simulink library "origionalPlant_cl"  (R2018b)
settings: Solver=VariableStepAuto  StartTime=0.0  StopTime=10.0  RelTol=1e-3
undefined symbols (not defined in the file or in its folder): X0
libraries: winch_ul x1
settings Model: Creator=mcobb  LastModifiedBy=mcobb

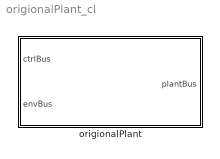
== system origionalPlant_cl ==
  origionalPlant : Subsystem  VariantControl=VSS_plant_origionalPlant

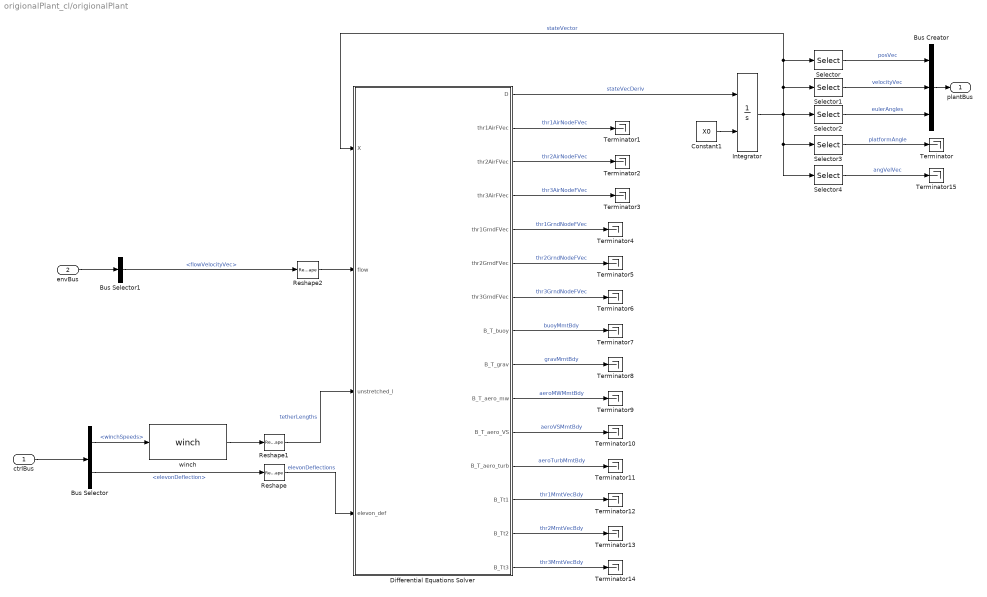
== system origionalPlant_cl/origionalPlant ==
  ctrlBus : Inport  OutDataTypeStr=Bus: ctrlBus
  envBus : Inport  Port=2  OutDataTypeStr=Bus: envBus
  Bus Creator : BusCreator  Inputs=3
  Bus Selector : BusSelector  OutputSignals=winchSpeeds,elevonDeflection
  Bus Selector1 : BusSelector  OutputSignals=flowVelocityVec
  Constant1 : Constant  Value=X0
  Differential Equations Solver : MATLAB Function  TreatAsAtomicUnit=on
  Integrator : Integrator  InitialConditionSource=external  InitialCondition=X0
  Reshape : Reshape  OutputDimensionality=Column vector (2-D)
  Reshape1 : Reshape  OutputDimensionality=Column vector (2-D)
  Reshape2 : Reshape  OutputDimensionality=Column vector (2-D)
  Selector : Selector  InputPortWidth=length(X0)  IndexOptions=Index vector (dialog)  Indices=[1 2 3]  OutputSizes=1
  Selector1 : Selector  InputPortWidth=length(X0)  IndexOptions=Index vector (dialog)  Indices=[4 5 6]  OutputSizes=1
  Selector2 : Selector  InputPortWidth=length(X0)  IndexOptions=Index vector (dialog)  Indices=[7 8 9]  OutputSizes=1
  Selector3 : Selector  InputPortWidth=length(X0)  IndexOptions=Index vector (dialog)  Indices=13  OutputSizes=1
  Selector4 : Selector  InputPortWidth=length(X0)  IndexOptions=Index vector (dialog)  Indices=[10 11 12]  OutputSizes=1
  Terminator{,1..15} (16 alike) : Terminator
  winch : winch_ul/winch  initLength=0  maxSpd=1  tau=0  maxAccl=1
  plantBus : Outport
  wires:
  Bus Selector/2 -> Reshape/1  "<elevonDeflection>"
  Bus Selector/1 -> winch/1  "<winchSpeeds>"
  Constant1/1 -> Integrator/2
  Differential Equations Solver/1(D) -> Integrator/1  "stateVecDeriv"
  Integrator/1 -> Differential Equations Solver/1(X), Selector/1, Selector1/1, Selector4/1, Selector3/1, Selector2/1  "stateVector"
  Selector1/1 -> Bus Creator/2  "velocityVec"
  Selector2/1 -> Bus Creator/3  "eulerAngles"
  Selector/1 -> Bus Creator/1  "posVec"
  Selector3/1 -> Terminator/1  "platformAngle"
  winch/1 -> Reshape1/1
  ctrlBus/1 -> Bus Selector/1
  envBus/1 -> Bus Selector1/1
  Bus Creator/1 -> plantBus/1
  Bus Selector1/1 -> Reshape2/1  "<flowVelocityVec>"
  Reshape/1 -> Differential Equations Solver/4(elevon_def)  "elevonDeflections"
  Reshape1/1 -> Differential Equations Solver/3(unstretched_l)  "tetherLengths"
  Reshape2/1 -> Differential Equations Solver/2(flow)
  Differential Equations Solver/2(thr1AirFVec) -> Terminator1/1  "thr1AirNodeFVec"
  Differential Equations Solver/7(thr3GrndFVec) -> Terminator6/1  "thr3GrndNodeFVec"
  Differential Equations Solver/6(thr2GrndFVec) -> Terminator5/1  "thr2GrndNodeFVec"
  Differential Equations Solver/5(thr1GrndFVec) -> Terminator4/1  "thr1GrndNodeFVec"
  Differential Equations Solver/4(thr3AirFVec) -> Terminator3/1  "thr3AirNodeFVec"
  Differential Equations Solver/3(thr2AirFVec) -> Terminator2/1  "thr2AirNodeFVec"
  Differential Equations Solver/15(B_Tt3) -> Terminator14/1  "thr3MmtVecBdy"
  Differential Equations Solver/14(B_Tt2) -> Terminator13/1  "thr2MmtVecBdy"
  Differential Equations Solver/13(B_Tt1) -> Terminator12/1  "thr1MmtVecBdy"
  Differential Equations Solver/12(B_T_aero_turb) -> Terminator11/1  "aeroTurbMmtBdy"
  Differential Equations Solver/11(B_T_aero_VS) -> Terminator10/1  "aeroVSMmtBdy"
  Differential Equations Solver/10(B_T_aero_mw) -> Terminator9/1  "aeroMWMmtBdy"
  Differential Equations Solver/9(B_T_grav) -> Terminator8/1  "gravMmtBdy"
  Differential Equations Solver/8(B_T_buoy) -> Terminator7/1  "buoyMmtBdy"
  Selector4/1 -> Terminator15/1  "angVelVec"

== matlab function origionalPlant_cl/origionalPlant/Differential Equations Solver ==
  data: X input size=size(X0); D output size=size(X0); flow input size=[3 1]; unstretched_l input size=[3 1]; elevon_def input size=[2 1]; sim_param parameter; thr1AirFVec output; thr2AirFVec output; thr3AirFVec output; thr1GrndFVec output; thr2GrndFVec output; thr3GrndFVec output; B_T_buoy output; B_T_grav output; B_T_aero_mw output; B_T_aero_VS output; B_T_aero_turb output; B_Tt1 output; B_Tt2 output; B_Tt3 output
 function [D,thr1AirFVec,thr2AirFVec,thr3AirFVec,thr1GrndFVec,thr2GrndFVec,...
     thr3GrndFVec,B_T_buoy,B_T_grav,B_T_aero_mw,B_T_aero_VS,B_T_aero_turb,B_Tt1,B_Tt2,B_Tt3]...
     = multimode_ode(X,flow,unstretched_l,elevon_def,sim_param)

D = zeros(size(X));

thr1AirFVec = [0 0 0]';
thr2AirFVec = [0 0 0]';
thr3AirFVec = [0 0 0]';
thr1GrndFVec = [0 0 0]';
thr2GrndFVec = [0 0 0]';
thr3GrndFVec = [0 0 0]';


B_T_buoy        = [0 0 0]';
B_T_grav        = [0 0 0]';
B_T_aero_mw     = [0 0 0]';
B_T_aero_VS     = [0 0 0]';
B_T_aero_turb   = [0 0 0]';
B_Tt1           = [0 0 0]';
B_Tt2           = [0 0 0]';
B_Tt3           = [0 0 0]';


%% number of nodes
N = sim_param.N;

% extract other values
mass = sim_param.geom_param.mass;
MI = sim_param.geom_param.MI;

P_Izz = sim_param.platform_param.platform_Izz;
cp = sim_param.platform_param.platform_damping;

R1n_cm = sim_param.tether_imp_nodes.R1n_cm;
R2n_cm = sim_param.tether_imp_nodes.R2n_cm;
R3n_cm = sim_param.tether_imp_nodes.R3n_cm;

R11_g = sim_param.tether_imp_nodes.R11_g;
R21_g = sim_param.tether_imp_nodes.R21_g;
R31_g = sim_param.tether_imp_nodes.R31_g;


%% constants
m = mass;
Ixx = MI(1,1);
Iyy = MI(2,2);
Izz = MI(3,3);

m_added = sim_param.geom_param.m_added;
Izz_added = sim_param.geom_param.Izz_added;

%% extract values from state space
% lifting body values
Rcm_o = X(1:3,1);
O_Vcm_o = X(4:6,1);

euler_ang = X(7:9,1);
    
ph = euler_ang(1);
th = euler_ang(2);
ps = euler_ang(3);

% rotations
[oCb,bCo] = rotation_sequence(euler_ang);

OwB = X(10:12,1);
wx = OwB(1);
wy = OwB(2);
wz = OwB(3);

psi_p = X(13,1);
platform_ang_vel = X(14,1);


pCo = [cos(psi_p) sin(psi_p) 0; -sin(psi_p) cos(psi_p) 0; 0 0 1];
oCp = pCo';


% tether position and velocity components
R1i_o = X(15:(14 + 3*N),1);
R2i_o = X((15 + 3*N):(14 + 6*N),1);
R3i_o = X((15 + 6*N):(14 + 9*N),1);

O_V1i_o = X((15 + 9*N):(14 + 12*N),1);
O_V2i_o = X((15 + 12*N):(14 + 15*N),1);
O_V3i_o = X((15 + 15*N):(14 + 18*N),1);


%%  center of mass first derivatives
D(1:3,1) = O_Vcm_o;
D(7,1) = wx + sin(ph)*tan(th)*wy + cos(ph)*tan(th)*wz;
D(8,1) = cos(ph)*wy - sin(ph)*wz;
D(9,1) = sec(th)*sin(ph)*wy + cos(ph)*sec(th)*wz;

%% platofrm angle first derivates
D(13,1) = platform_ang_vel;
OwP = [0;0;platform_ang_vel];

%% grnd station first derivative
D(15:17,1) = [0;0;0];

%% changing first node first deivative
O_V1i_o(1:3,1) = oCp*(cross(OwP,R11_g));
O_V2i_o(1:3,1) = oCp*(cross(OwP,R21_g));
O_V3i_o(1:3,1) = oCp*(cross(OwP,R31_g));

%% changing last node first deivative
O_V1i_o((end-2):end,1) = O_Vcm_o + oCb*(cross(OwB,R1n_cm));
O_V2i_o((end-2):end,1)=  O_Vcm_o + oCb*(cross(OwB,R2n_cm));
O_V3i_o((end-2):end,1)=  O_Vcm_o + oCb*(cross(OwB,R3n_cm));

%% tether nodes first derivatives
D(15:(14 + 3*N),1) = O_V1i_o;
D((15 + 3*N):(14 + 6*N),1) = O_V2i_o;
D((15 + 6*N):(14 + 9*N),1) = O_V3i_o;


%% EXTERNAL FORCES AND TORQUES
op = multinode_F_and_T_external(sim_param,flow,unstretched_l,elevon_def,Rcm_o,R1i_o,R2i_o,R3i_o,...
    O_Vcm_o,O_V1i_o,O_V2i_o,O_V3i_o,OwB,euler_ang,psi_p);

O_F_ext = op.O_F_ext;
B_T_ext = op.B_T_ext;
sum_1_f = op.sum_1_f;
sum_2_f = op.sum_2_f;
sum_3_f = op.sum_3_f;
T_o_ext = op.T_o_ext;

if any(abs(O_F_ext)>10^6) || any(abs(B_T_ext)>10^6) || any(any(abs(sum_1_f)>10^6)) || any(any(abs(sum_2_f)>10^6)) || any(any(abs(sum_3_f)>10^6))
    x = 1;
end


Tx = B_T_ext(1);
Ty = B_T_ext(2);
Tz = B_T_ext(3);

% mass at each node
tether_masses = op.tether_masses;

m1i = tether_masses(1)/(N-2);
m2i = tether_masses(2)/(N-2);
m3i = tether_masses(3)/(N-2);

%% center of mass second derivatives
% added mass
mass_matrix = [1/(m+m_added(1)) 0 0;0 1/(m+m_added(2)) 0;0 0 1/(m+m_added(3))];

D(4:6,1) = oCb*(mass_matrix*(bCo*O_F_ext));
D(10,1) = (1/Ixx)*(Tx + (Iyy - Izz)*wy*wz);
D(11,1) = (1/Iyy)*(Ty + (Izz - Ixx)*wx*wz);
D(12,1) = (1/(Izz+Izz_added))*(Tz + (Ixx - Iyy)*wx*wy);

OaB = D(10:12,1);

%% platform angle second derivative
% D(14,1) = (T_o_ext/P_Izz) - cp*platform_ang_vel; % Origional
D(14,1) = 0; % Zero rotation
if sim_param.freeSpinPlatform
    D(14,1) = (T_o_ext - cp*platform_ang_vel)/P_Izz; % Corrected
else
    
% 

OaP = [0;0;D(14,1)];

%% tether nodes 2nd derivatives

for i = 1:N
    
    if i == 1 
        D((14 + 9*N + 3*i - 2):(14 + 9*N + 3*i),1) = oCp*( cross(OaP,R11_g) +  cross(OwP,(cross(OwP,R11_g))) );
        D((14 + 12*N + 3*i - 2):(14 + 12*N + 3*i),1) = oCp*( cross(OaP,R21_g) +  cross(OwP,(cross(OwP,R21_g))) );
        D((14 + 15*N + 3*i - 2):(14 + 15*N + 3*i),1) = oCp*( cross(OaP,R31_g) +  cross(OwP,(cross(OwP,R31_g))) );
   
    elseif i>1 && i<N
        if any(any(sum_1_f))>10^10
           x = 1; 
        end
        D((14 + 9*N + 3*i - 2):(14 + 9*N + 3*i),1) = (1/m1i)*sum_1_f(:,i);
        D((14 + 12*N + 3*i - 2):(14 + 12*N + 3*i),1) = (1/m2i)*sum_2_f(:,i);
        D((14 + 15*N + 3*i - 2):(14 + 15*N + 3*i),1) = (1/m3i)*sum_3_f(:,i);
        
    elseif i == N
        
        D((14 + 9*N + 3*i - 2):(14 + 9*N + 3*i),1) = D(4:6,1) + ...
            oCb*( cross(OaB,R1n_cm) +  cross(OwB,(cross(OwB,R1n_cm))) );
        
        
        D((14 + 12*N + 3*i - 2):(14 + 12*N + 3*i),1) =  D(4:6,1) + ...
            oCb*( cross(OaB,R2n_cm) +  cross(OwB,(cross(OwB,R2n_cm))) ) ;
        
        D((14 + 15*N + 3*i - 2):(14 + 15*N + 3*i),1) =  D(4:6,1) + ...
            oCb*( cross(OaB,R3n_cm) +  cross(OwB,(cross(OwB,R3n_cm))) );
        
    end
    
    
end



thr1AirFVec = sum_1_f(:,end);
thr2AirFVec = sum_2_f(:,end);
thr3AirFVec = sum_3_f(:,end);
thr1GrndFVec = sum_1_f(:,1);
thr2GrndFVec = sum_2_f(:,1);
thr3GrndFVec = sum_3_f(:,1);

B_T_buoy        = op.B_T_buoy;
B_T_grav        = op.B_T_grav;
B_T_aero_mw     = op.B_T_aero_mw;
B_T_aero_VS     = op.B_T_aero_VS;
B_T_aero_turb   = op.B_T_aero_turb;
B_Tt1           = op.B_Tt1;
B_Tt2           = op.B_Tt2;
B_Tt3           = op.B_Tt3;



 end
